simulink model "sliderSim"  (R2025b)
settings: Solver=VariableStepAuto  StartTime=0.0  StopTime=simTime  RelTol=1e-3
values from neighbouring files (symbols this model uses):
  failureTime = 0    [simSetup.m]
  healthy = bin2dec('10011111') + 1    [simSetup.m]
  I_zz = 1.092    [simSetup.m]
  init = [3 0 0 0 0 0]    [simSetup.m]
  Kd = diag([8 8 1.2])    [simSetup.m]
  ki = diag([0.05 0.05 0.064])    [simSetup.m]
  Kp = diag([2 2 0.48])    [simSetup.m]
  mass = 4.436    [simSetup.m]
  ref = [3,5,0,0,0,0]'    [simSetup.m]
settings Model: Creator=glim  LastModifiedBy=glim

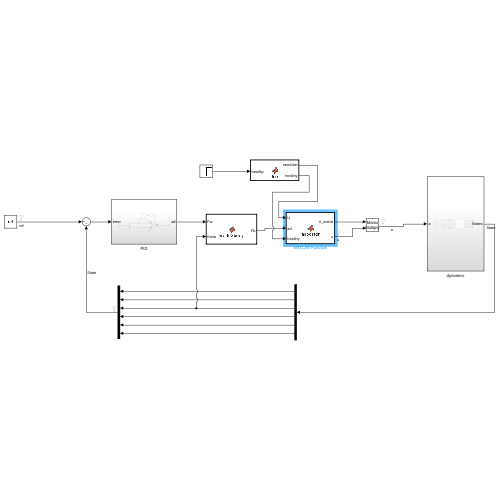
[thumbnail: Simulink's stored preview of the top-level diagram]
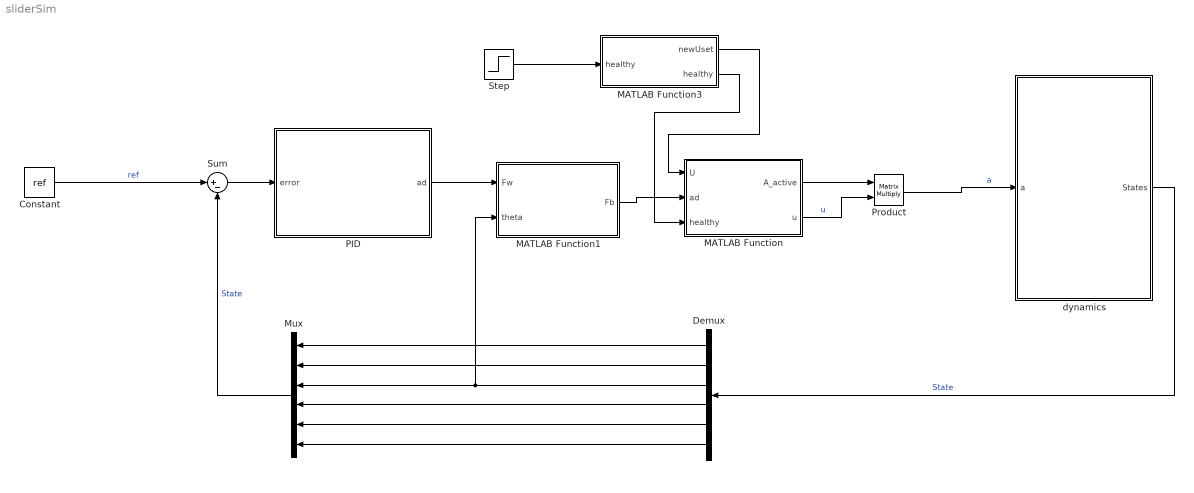
== system sliderSim ==
  Constant : Constant  Value=ref  VectorParams1D=off
  Demux : Demux  Outputs=6
  MATLAB Function : MATLAB Function  TreatAsAtomicUnit=on
  MATLAB Function1 : MATLAB Function  TreatAsAtomicUnit=on
  MATLAB Function3 : MATLAB Function  TreatAsAtomicUnit=on
  Mux : Mux  Inputs=6
  PID : Subsystem
  Product : Product  Multiplication=Matrix(*)
  Step : Step  Time=failureTime  Before=256  After=healthy  SampleTime=0
  Sum : Sum  Inputs=|+-
  dynamics : Subsystem
  wires:
  Constant/1 -> Sum/1  "ref"
  Sum/1 -> PID/1(error)
  PID/1(ad) -> MATLAB Function1/1(Fw)
  MATLAB Function1/1(Fb) -> MATLAB Function/2(ad)
  dynamics/1(States) -> Demux/1  "State"
  Demux/1 -> Mux/1
  Demux/2 -> Mux/2
  Demux/3 -> MATLAB Function1/2(theta), Mux/3
  Demux/4 -> Mux/4
  Demux/5 -> Mux/5
  Demux/6 -> Mux/6
  Mux/1 -> Sum/2  "State"
  Step/1 -> MATLAB Function3/1("healthy ")
  MATLAB Function3/2(healthy) -> MATLAB Function/3(healthy)
  MATLAB Function3/1(newUset) -> MATLAB Function/1(U)
  MATLAB Function/1(A_active) -> Product/1
  MATLAB Function/2(u) -> Product/2  "u"
  Product/1 -> dynamics/1(a)  "a"

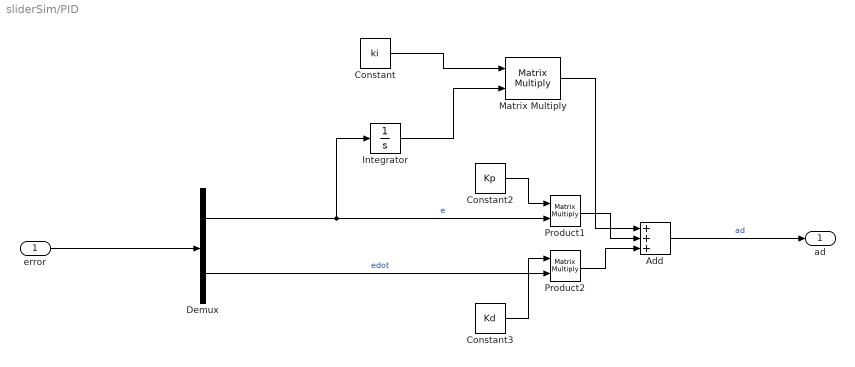
== system sliderSim/PID ==
  error : Inport
  Add : Sum  Inputs=+++
  Constant : Constant  Value=ki  VectorParams1D=off
  Constant2 : Constant  Value=Kp
  Constant3 : Constant  Value=Kd
  Demux : Demux  Outputs=2
  Integrator : Integrator
  Matrix Multiply : Product  Multiplication=Matrix(*)
  Product1 : Product  Multiplication=Matrix(*)
  Product2 : Product  Multiplication=Matrix(*)
  ad : Outport
  wires:
  Demux/1 -> Integrator/1, Product1/2  "e"
  Constant2/1 -> Product1/1
  Demux/2 -> Product2/2  "edot"
  Constant3/1 -> Product2/1
  error/1 -> Demux/1
  Add/1 -> ad/1  "ad"
  Integrator/1 -> Matrix Multiply/2
  Constant/1 -> Matrix Multiply/1
  Product2/1 -> Add/3
  Product1/1 -> Add/2
  Matrix Multiply/1 -> Add/1

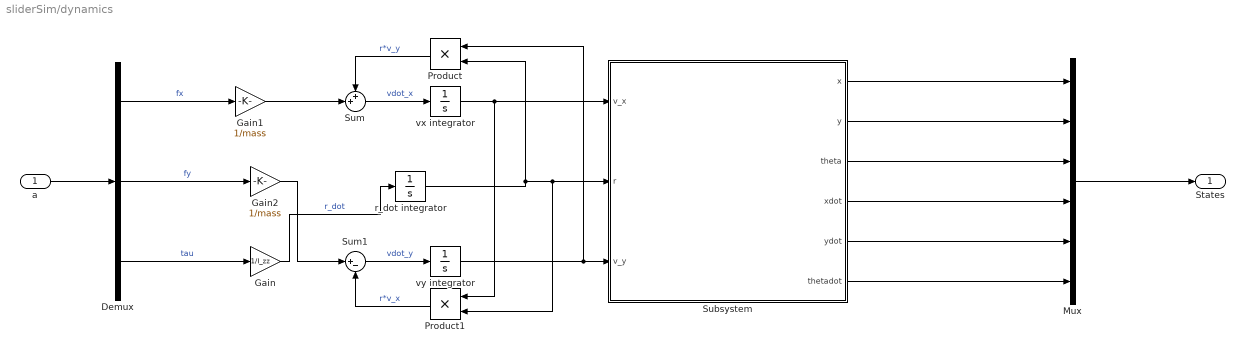
== system sliderSim/dynamics ==
  a : Inport
  Demux : Demux  Outputs=3
  Gain : Gain  Gain=1/I_zz
  Gain1 : Gain  Gain=1/mass
  Gain2 : Gain  Gain=1/mass
  Mux : Mux  Inputs=6
  Product : Product
  Product1 : Product
  Subsystem : Subsystem
  Sum : Sum  Inputs=++|
  Sum1 : Sum  Inputs=|+-
  r_dot integrator : Integrator  InitialCondition=init(6)
  vx integrator : Integrator  InitialCondition=init(4)  ContinuousStateAttributes='vx'
  vy integrator : Integrator  InitialCondition=init(5)
  States : Outport
  wires:
  Product/1 -> Sum/1  "r*v_y"
  Product1/1 -> Sum1/2  "r*v_x"
  vy integrator/1 -> Product/1, Subsystem/3(v_y)
  vx integrator/1 -> Product1/1, Subsystem/1(v_x)
  Gain1/1 -> Sum/2
  Sum1/1 -> vy integrator/1  "vdot_y"
  Sum/1 -> vx integrator/1  "vdot_x"
  Gain/1 -> r_dot integrator/1  "r_dot"
  r_dot integrator/1 -> Product/2, Subsystem/2(r), Product1/2
  Gain2/1 -> Sum1/1
  Demux/1 -> Gain1/1  "fx"
  a/1 -> Demux/1
  Demux/2 -> Gain2/1  "fy"
  Demux/3 -> Gain/1  "tau"
  Subsystem/5(ydot) -> Mux/5
  Subsystem/4(xdot) -> Mux/4
  Subsystem/3(theta) -> Mux/3
  Subsystem/1(x) -> Mux/1
  Subsystem/6(thetadot) -> Mux/6
  Mux/1 -> States/1
  Subsystem/2(y) -> Mux/2

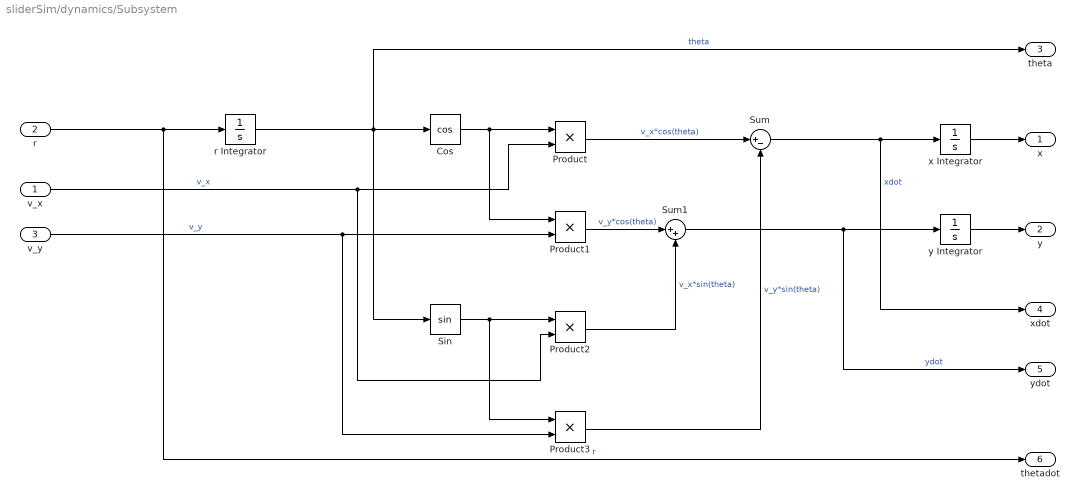
== system sliderSim/dynamics/Subsystem ==
  v_x : Inport
  r : Inport  Port=2
  v_y : Inport  Port=3
  Cos : Trigonometry  Operator=cos
  Product{,1..3} (4 alike) : Product
  Sin : Trigonometry
  Sum : Sum  Inputs=|+-
  Sum1 : Sum  Inputs=|++
  r Integrator : Integrator  InitialCondition=init(3)
  x Integrator : Integrator  InitialCondition=init(1)
  y Integrator : Integrator  InitialCondition=init(2)
  x : Outport
  y : Outport  Port=2
  theta : Outport  Port=3
  xdot : Outport  Port=4
  ydot : Outport  Port=5
  thetadot : Outport  Port=6
  wires:
  r Integrator/1 -> theta/1, Sin/1, Cos/1  "theta"
  Cos/1 -> Product1/1, Product/1
  v_x/1 -> Product/2, Product2/2  "v_x"
  Product/1 -> Sum/1  "v_x*cos(theta)"
  v_y/1 -> Product3/2, Product1/2  "v_y"
  Product1/1 -> Sum1/1  "v_y*cos(theta)"
  Sin/1 -> Product3/1, Product2/1
  Product2/1 -> Sum1/2  "v_x*sin(theta)"
  Product3/1 -> Sum/2  "v_y*sin(theta)"
  Sum/1 -> xdot/1, x Integrator/1  "xdot"
  x Integrator/1 -> x/1
  Sum1/1 -> ydot/1, y Integrator/1  "ydot"
  y Integrator/1 -> y/1
  r/1 -> thetadot/1, r Integrator/1  "r"

== matlab function sliderSim/MATLAB Function1 ==
  data: Fw input; Fb output; theta input
function Fb = world2body(Fw, theta)
    % Fw = [Fx_w; Fy_w; tau_w], Fb = [Fx_b; Fy_b; tau_b]
    c = cos(theta); s = sin(theta);
    Fx_b =  c*Fw(1) + s*Fw(2);
    Fy_b = -s*Fw(1) + c*Fw(2);
    tau_b = Fw(3);
    Fb = [Fx_b; Fy_b; tau_b];
end

== matlab function sliderSim/MATLAB Function ==
  settings: updateMethod=DISCRETE
  data: A_active output size=[3 8]; U input; ad input size=[3 1]; u output size=[8 1]; healthy input; uCache parameter size=[1, 256]
function [A_active,u] = allocator(U,ad,healthy,uCache)

    A_active = uCache(healthy).A;
    [u, ~, ~] = findUfromAd_DA(ad,U, A_active);
end

== matlab function sliderSim/MATLAB Function3 ==
  data: healthy input; newUset output size=[8 4 56] [1176..1792]; uCache parameter size=[1, 256]; healthy output size=[1]
function [newUset, healthy] = fcn(healthy,uCache)
    newUset = uCache(healthy).U;
end
